simulink model "non_linear"  (R2016a)
settings: Solver=FixedStepAuto  StartTime=0.0  StopTime=300  FixedStep=0.0005  RelTol=1e-3
libraries: simulink x3
settings Model: Creator=mikae  LastModifiedBy=jamie

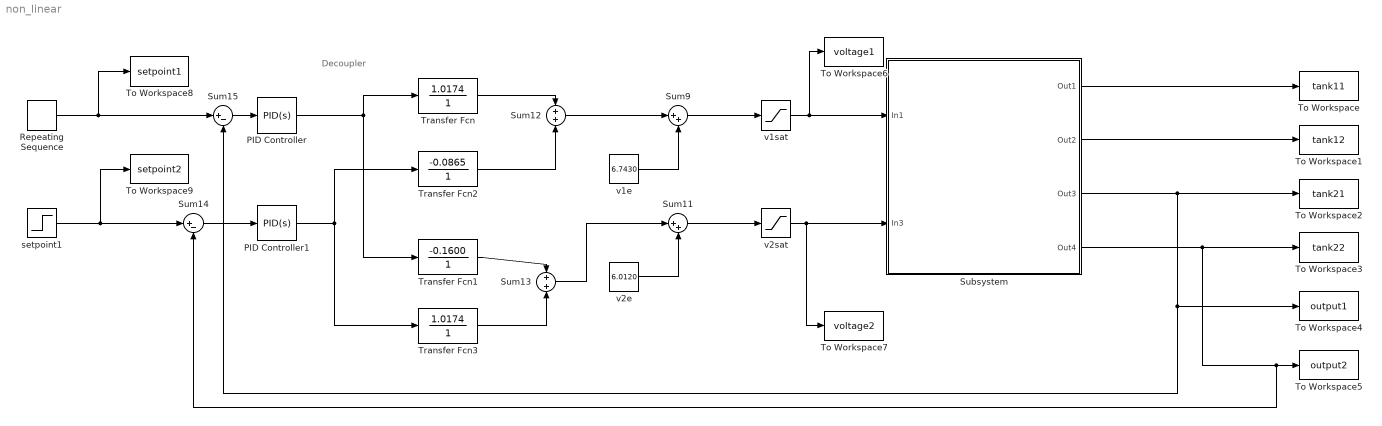
== system non_linear ==
  note: Decoupler
  PID Controller : simulink/Continuous/PID Controller  Controller=PID  TimeDomain=Continuous-time  SampleTime=-1  IntegratorMethod=Forward Euler  FilterMethod=Forward Euler  Form=Ideal  UseFilter=on  ControllerParametersSource=internal  P=1.4351  I=0.0051437  D=10.0105  N=100  InitialConditionSource=internal  InitialConditionForIntegrator=0  InitialConditionForFilter=0  ExternalReset=none  LimitOutput=off  UpperSaturationLimit=inf  LowerSaturationLimit=-inf  LinearizeAsGain=on  AntiWindupMode=none  Kb=1  TrackingMode=off  Kt=1  PParamMin=[]  PParamMax=[]  IParamMin=[]  IParamMax=[]  DParamMin=[]  DParamMax=[]  NParamMin=[]  NParamMax=[]  KbParamMin=[]  KbParamMax=[]  KtParamMin=[]  KtParamMax=[]  POutMin=[]  POutMax=[]  IOutMin=[]  IOutMax=[]  DOutMin=[]  DOutMax=[]  NOutMin=[]  NOutMax=[]  KbOutMin=[]  KbOutMax=[]  KtOutMin=[]  KtOutMax=[]  IntegratorOutMin=[]  IntegratorOutMax=[]  FilterOutMin=[]  FilterOutMax=[]  SumOutMin=[]  SumOutMax=[]  SumI1OutMin=[]  SumI1OutMax=[]  SumI2OutMin=[]  SumI2OutMax=[]  SumI3OutMin=[]  SumI3OutMax=[]  SumDOutMin=[]  SumDOutMax=[]  SaturationOutMin=[]  SaturationOutMax=[]  IntegratorContinuousStateAttributes=''  IntegratorStateMustResolveToSignalObject=off  IntegratorRTWStateStorageClass=Auto  FilterContinuousStateAttributes=''  FilterStateMustResolveToSignalObject=off  FilterRTWStateStorageClass=Auto  DifferentiatorICPrevScaledInput=0  DifferentiatorOutMin=[]  DifferentiatorOutMax=[]
  PID Controller1 : simulink/Continuous/PID Controller  Controller=PID  TimeDomain=Continuous-time  SampleTime=-1  IntegratorMethod=Forward Euler  FilterMethod=Forward Euler  Form=Parallel  UseFilter=on  ControllerParametersSource=internal  P=1.4351  I=0.0051437  D=10.0105  N=100  InitialConditionSource=internal  InitialConditionForIntegrator=0  InitialConditionForFilter=0  ExternalReset=none  LimitOutput=off  UpperSaturationLimit=inf  LowerSaturationLimit=-inf  LinearizeAsGain=on  AntiWindupMode=none  Kb=1  TrackingMode=off  Kt=1  PParamMin=[]  PParamMax=[]  IParamMin=[]  IParamMax=[]  DParamMin=[]  DParamMax=[]  NParamMin=[]  NParamMax=[]  KbParamMin=[]  KbParamMax=[]  KtParamMin=[]  KtParamMax=[]  POutMin=[]  POutMax=[]  IOutMin=[]  IOutMax=[]  DOutMin=[]  DOutMax=[]  NOutMin=[]  NOutMax=[]  KbOutMin=[]  KbOutMax=[]  KtOutMin=[]  KtOutMax=[]  IntegratorOutMin=[]  IntegratorOutMax=[]  FilterOutMin=[]  FilterOutMax=[]  SumOutMin=[]  SumOutMax=[]  SumI1OutMin=[]  SumI1OutMax=[]  SumI2OutMin=[]  SumI2OutMax=[]  SumI3OutMin=[]  SumI3OutMax=[]  SumDOutMin=[]  SumDOutMax=[]  SaturationOutMin=[]  SaturationOutMax=[]  IntegratorContinuousStateAttributes=''  IntegratorStateMustResolveToSignalObject=off  IntegratorRTWStateStorageClass=Auto  FilterContinuousStateAttributes=''  FilterStateMustResolveToSignalObject=off  FilterRTWStateStorageClass=Auto  DifferentiatorICPrevScaledInput=0  DifferentiatorOutMin=[]  DifferentiatorOutMax=[]
  Repeating Sequence : simulink/Sources/Repeating Sequence  rep_seq_t="[1\t1.50000000000000\t2\t2.50000000000000\t3\t3.50000000000000\t4\t4.50000000000000\t5\t5.50000000000000\t6\t6.50000000000000\t7\t7.50000000000000\t8\t8.50000000000000\t9\t9.50000000000000\t10\t10.5000000000000\t11\t11.5000000000000\t12\t12.5000000000000\t13\t13.5000000000000\t14\t14.5000000000000\t15\t15.5000000000000\t16\t16.5000000000000\t17\t17.5000000000000\t18\t18.5000000000000\t19\t19.5000000000000\t20\t20.5000000000000\t21\t21.5000000000000\t22\t22.5000000000000\t23\t23.5000000000000\t24\t24.5000000000000\t25\t25.5000000000000\t26\t26.5000000000000\t27\t27.5000000000000\t28\t28.5000000000000\t29\t29.5000000000000\t30\t30.5000000000000\t31\t31.5000000000000\t32\t32.5000000000000\t33\t33.5000000000000\t34\t34.5000000000000\t35\t35.5000000000000\t36\t36.5000000000000\t37\t37.5000000000000\t38\t38.5000000000000\t39\t39.5000000000000\t40\t40.5000000000000\t41\t41.5000000000000\t42\t42.5000000000000\t43\t43.5000000000000\t44\t44.5000000000000\t45\t45.5000000000000\t46\t46.5000000000000\t47\t47.5000000000000\t48\t48.5000000000000\t49\t49.5000000000000\t50\t50.5000000000000\t51\t51.5000000000000\t52\t52.5000000000000\t53\t53.5000000000000\t54\t54.5000000000000\t55\t55.5000000000000\t56\t56.5000000000000\t57\t57.5000000000000\t58\t58.5000000000000\t59\t59.5000000000000\t60\t60.5000000000000\t61\t61.5000000000000\t62\t62.5000000000000\t63\t63.5000000000000\t64\t64.5000000000000\t65\t65.5000000000000\t66\t66.5000000000000\t67\t67.5000000000000\t68\t68.5000000000000\t69\t69.5000000000000\t70\t70.5000000000000\t71\t71.5000000000000\t72\t72.5000000000000\t73\t73.5000000000000\t74\t74.5000000000000\t75\t75.5000000000000\t76\t76.5000000000000\t77\t77.5000000000000\t78\t78.5000000000000\t79\t79.5000000000000\t80\t80.5000000000000\t81\t81.5000000000000\t82\t82.5000000000000\t83\t83.5000000000000\t84\t84.5000000000000\t85\t85.5000000000000\t86\t86.5000000000000\t87\t87.5000000000000\t88\t88.5000000000000\t89\t89.5000000000000\t90\t90.5000000000000\t91\t91.5000000000000\t92\t92.5000000000000\t93\t93.5000000000000\t94\t94.5000000000000\t95\t95.5000000000000\t96\t96.5000000000000\t97\t97.5000000000000\t98\t98.5000000000000\t99\t99.5000000000000\t100\t100.500000000000\t101\t101.500000000000\t102\t102.500000000000\t103\t103.500000000000\t104\t104.500000000000\t105\t105.500000000000\t106\t106.500000000000\t107\t107.500000000000\t108\t108.500000000000\t109\t109.500000000000\t110\t110.500000000000\t111\t111.500000000000\t112\t112.500000000000\t113\t113.500000000000\t114\t114.500000000000\t115\t115.500000000000\t116\t116.500000000000\t117\t117.500000000000\t118\t118.500000000000\t119\t119.500000000000\t120\t120.500000000000\t121\t121.500000000000\t122\t122.500000000000\t123\t123.500000000000\t124\t124.500000000000\t125\t125.500000000000\t126\t126.500000000000\t127\t127.500000000000\t128\t128.500000000000\t129\t129.500000000000\t130\t130.500000000000\t131\t131.500000000000\t132\t132.500000000000\t133\t133.500000000000\t134\t134.500000000000\t135\t135.500000000000\t136\t136.500000000000\t137\t137.500000000000\t138\t138.500000000000\t139\t139.500000000000\t140\t140.500000000000\t141\t141.500000000000\t142\t142.500000000000\t143\t143.500000000000\t144\t144.500000000000\t145\t145.500000000000\t146\t146.500000000000\t147\t147.500000000000\t148\t148.500000000000\t149\t149.500000000000\t150\t150.500000000000\t151\t151.500000000000\t152\t152.500000000000\t153\t153.500000000000\t154\t154.500000000000\t155\t155.500000000000\t156\t156.500000000000\t157\t157.500000000000\t158\t158.500000000000\t159\t159.500000000000\t160\t160.500000000000\t161\t161.500000000000\t162\t162.500000000000\t163\t163.500000000000\t164\t164.500000000000\t165\t165.500000000000\t166\t166.500000000000\t167\t167.500000000000\t168\t168.500000000000\t169\t169.500000000000\t170\t170.500000000000\t171\t171.500000000000\t172\t172.500000000000\t173\t173.500000000000\t174\t174.500000000000\t175\t175.500000000000\t176\t176.500000000000\t177\t177.500000000000\t178\t178.500000000000\t179\t179.500000000000\t180\t180.500000000000\t181\t181.500000000000\t182\t182.500000000000\t183\t183.500000000000\t184\t184.500000000000\t185\t185.500000000000\t186\t186.500000000000\t187\t187.500000000000\t188\t188.500000000000\t189\t189.500000000000\t190\t190.500000000000\t191\t191.500000000000\t192\t192.500000000000\t193\t193.500000000000\t194\t194.500000000000\t195\t195.500000000000\t196\t196.500000000000\t197\t197.500000000000\t198\t198.500000000000\t199\t199.500000000000\t200\t200.500000000000\t201\t201.500000000000\t202\t202.500000000000\t203\t203.500000000000\t204\t204.500000000000\t205\t205.500000000000\t206\t206.500000000000\t207\t207.500000000000\t208\t208.500000000000\t209\t209.500000000000\t210\t210.500000000000\t211\t211.500000000000\t212\t212.500000000000\t213\t213.500000000000\t214\t214.500000000000\t215\t215.500000000000\t216\t216.500000000000\t217\t217.500000000000\t218\t218.500000000000\t219\t219.500000000000\t220\t220.500000000000\t221\t221.500000000000\t222\t222.500000000000\t223\t223.500000000000\t224\t224.500000000000\t225\t225.500000000000\t226\t226.500000000000\t227\t227.500000000000\t228\t228.500000000000\t229\t229.500000000000\t230\t230.500000000000\t231\t231.500000000000\t232\t232.500000000000\t233\t233.500000000000\t234\t234.500000000000\t235\t235.500000000000\t236\t236.500000000000\t237\t237.500000000000\t238\t238.500000000000\t239\t239.500000000000\t240\t240.500000000000\t241\t241.500000000000\t242\t242.500000000000\t243\t243.500000000000\t244\t244.500000000000\t245\t245.500000000000\t246\t246.500000000000\t247\t247.500000000000\t248\t248.500000000000\t249\t249.500000000000\t250\t250.500000000000]"  rep_seq_y="[2\t2\t2\t2\t2\t2\t2\t2\t2\t2\t2\t2\t2\t2\t2\t2\t2\t2\t2\t2\t2\t2\t2\t2\t2\t2\t2\t2\t2\t2\t2\t2\t2\t2\t2\t2\t2\t2\t2\t2\t2\t2\t2\t2\t2\t2\t2\t2\t2\t2\t2\t2\t2\t2\t2\t2\t2\t2\t2\t2\t2\t2\t2\t2\t2\t2\t2\t2\t2\t2\t2\t2\t2\t2\t2\t2\t2\t2\t2\t2\t2\t2\t2\t2\t2\t2\t2\t2\t2\t2\t2\t2\t2\t2\t2\t2\t2\t2\t2\t2\t2.10800000000000\t2.21600000000000\t2.32400000000000\t2.43200000000000\t2.54000000000000\t2.64800000000000\t2.75600000000000\t2.86400000000000\t2.97200000000000\t3.08000000000000\t3.18800000000000\t3.29600000000000\t3.40400000000000\t3.51200000000000\t3.62000000000000\t3.72800000000000\t3.83600000000000\t3.94400000000000\t4.05200000000000\t4.16000000000000\t4.26800000000000\t4.37600000000000\t4.48400000000000\t4.59200000000000\t4.70000000000000\t4.80800000000000\t4.91600000000000\t5.02400000000000\t5.13200000000000\t5.24000000000000\t5.34800000000000\t5.45600000000000\t5.56400000000000\t5.67200000000000\t5.78000000000000\t5.88800000000000\t5.99600000000000\t6.10400000000000\t6.21200000000000\t6.32000000000000\t6.42800000000000\t6.53600000000000\t6.64400000000000\t6.75200000000000\t6.86000000000000\t6.96800000000000\t7.07600000000000\t7.18400000000000\t7.29200000000000\t7.40000000000000\t7.50800000000000\t7.61600000000000\t7.72400000000000\t7.83200000000000\t7.94000000000000\t8.04800000000000\t8.15600000000000\t8.26400000000000\t8.37200000000000\t8.48000000000000\t8.58800000000000\t8.69600000000000\t8.80400000000000\t8.91200000000000\t9.02000000000000\t9.12800000000000\t9.23600000000000\t9.34400000000000\t9.45200000000000\t9.56000000000000\t9.66800000000000\t9.77600000000000\t9.88400000000000\t9.99200000000000\t10.1000000000000\t10.2080000000000\t10.3160000000000\t10.4240000000000\t10.5320000000000\t10.6400000000000\t10.7480000000000\t10.8560000000000\t10.9640000000000\t11.0720000000000\t11.1800000000000\t11.2880000000000\t11.3960000000000\t11.5040000000000\t11.6120000000000\t11.7200000000000\t11.8280000000000\t11.9360000000000\t12.0440000000000\t12.1520000000000\t12.2600000000000\t12.3680000000000\t12.4760000000000\t12.5840000000000\t12.6920000000000\t12.8000000000000\t12.9080000000000\t13.0160000000000\t13.1240000000000\t13.2320000000000\t13.3400000000000\t13.4480000000000\t13.5560000000000\t13.6640000000000\t13.7720000000000\t13.8800000000000\t13.9880000000000\t14.0960000000000\t14.2040000000000\t14.3120000000000\t14.4200000000000\t14.5280000000000\t14.6360000000000\t14.7440000000000\t14.8520000000000\t14.9600000000000\t15.0680000000000\t15.1760000000000\t15.2840000000000\t15.3920000000000\t15.5000000000000\t15.5000000000000\t15.5000000000000\t15.5000000000000\t15.5000000000000\t15.5000000000000\t15.5000000000000\t15.5000000000000\t15.5000000000000\t15.5000000000000\t15.5000000000000\t15.5000000000000\t15.5000000000000\t15.5000000000000\t15.5000000000000\t15.5000000000000\t15.5000000000000\t15.5000000000000\t15.5000000000000\t15.5000000000000\t15.5000000000000\t15.5000000000000\t15.5000000000000\t15.5000000000000\t15.5000000000000\t15.5000000000000\t15.5000000000000\t15.5000000000000\t15.5000000000000\t15.5000000000000\t15.5000000000000\t15.5000000000000\t15.5000000000000\t15.5000000000000\t15.5000000000000\t15.5000000000000\t15.5000000000000\t15.5000000000000\t15.5000000000000\t15.5000000000000\t15.5000000000000\t15.5000000000000\t15.5000000000000\t15.5000000000000\t15.5000000000000\t15.5000000000000\t15.5000000000000\t15.5000000000000\t15.5000000000000\t15.5000000000000\t15.5000000000000\t15.5000000000000\t15.5000000000000\t15.5000000000000\t15.5000000000000\t15.5000000000000\t15.5000000000000\t15.5000000000000\t15.5000000000000\t15.5000000000000\t15.5000000000000\t15.5000000000000\t15.5000000000000\t15.5000000000000\t15.5000000000000\t15.5000000000000\t15.5000000000000\t15.5000000000000\t15.5000000000000\t15.5000000000000\t15.5000000000000\t15.5000000000000\t15.5000000000000\t15.5000000000000\t15.5000000000000\t15.5000000000000\t15.5000000000000\t15.5000000000000\t15.5000000000000\t15.5000000000000\t15.5000000000000\t15.5000000000000\t15.5000000000000\t15.5000000000000\t15.5000000000000\t15.5000000000000\t15.5000000000000\t15.5000000000000\t15.5000000000000\t15.5000000000000\t15.5000000000000\t15.6180000000000\t15.7360000000000\t15.8540000000000\t15.9720000000000\t16.0900000000000\t16.2080000000000\t16.3260000000000\t16.4440000000000\t16.5620000000000\t16.6800000000000\t16.7980000000000\t16.9160000000000\t17.0340000000000\t17.1520000000000\t17.2700000000000\t17.3880000000000\t17.5060000000000\t17.6240000000000\t17.7420000000000\t17.8600000000000\t17.9780000000000\t18.0960000000000\t18.2140000000000\t18.3320000000000\t18.4500000000000\t18.5680000000000\t18.6860000000000\t18.8040000000000\t18.9220000000000\t19.0400000000000\t19.1580000000000\t19.2760000000000\t19.3940000000000\t19.5120000000000\t19.6300000000000\t19.7480000000000\t19.8660000000000\t19.9840000000000\t20.1020000000000\t20.2200000000000\t20.3380000000000\t20.4560000000000\t20.5740000000000\t20.6920000000000\t20.8100000000000\t20.9280000000000\t21.0460000000000\t21.1640000000000\t21.2820000000000\t21.4000000000000\t21.5180000000000\t21.6360000000000\t21.7540000000000\t21.8720000000000\t21.9900000000000\t21.8850000000000\t21.7700000000000\t21.6550000000000\t21.5400000000000\t21.4250000000000\t21.3100000000000\t21.1950000000000\t21.0800000000000\t20.9650000000000\t20.8500000000000\t20.7350000000000\t20.6200000000000\t20.5050000000000\t20.3900000000000\t20.2750000000000\t20.1600000000000\t20.0450000000000\t19.9300000000000\t19.8150000000000\t19.7000000000000\t19.5850000000000\t19.4700000000000\t19.3550000000000\t19.2400000000000\t19.1250000000000\t19.0100000000000\t18.8950000000000\t18.7800000000000\t18.6650000000000\t18.5500000000000\t18.4350000000000\t18.3200000000000\t18.2050000000000\t18.0900000000000\t17.9750000000000\t17.8600000000000\t17.7450000000000\t17.6300000000000\t17.5150000000000\t17.4000000000000\t17.2850000000000\t17.1700000000000\t17.0550000000000\t16.9400000000000\t16.8250000000000\t16.7100000000000\t16.5950000000000\t16.4800000000000\t16.3650000000000\t16.2500000000000\t16.1350000000000\t16.0200000000000\t15.9050000000000\t15.7900000000000\t15.6750000000000\t15.5600000000000\t15.4450000000000\t15.3300000000000\t15.2150000000000\t15.1000000000000\t14.9850000000000\t14.8700000000000\t14.7550000000000\t14.6400000000000\t14.5250000000000\t14.4100000000000\t14.2950000000000\t14.1800000000000\t14.0650000000000\t13.9500000000000\t13.8350000000000\t13.7200000000000\t13.6050000000000\t13.4900000000000\t13.3750000000000\t13.2600000000000\t13.1450000000000\t13.0300000000000\t12.9150000000000\t12.8000000000000\t12.6850000000000\t12.5700000000000\t12.4550000000000\t12.3400000000000\t12.2250000000000\t12.1100000000000\t11.9950000000000\t11.8800000000000\t11.7650000000000\t11.6500000000000\t11.5350000000000\t11.4200000000000\t11.3050000000000\t11.1900000000000\t11.0750000000000\t10.9600000000000\t10.8450000000000\t10.7300000000000\t10.6150000000000\t10.5000000000000\t10.3850000000000\t10.2700000000000\t10.1550000000000\t10.0400000000000\t9.92500000000000\t9.81000000000000\t9.69500000000000\t9.58000000000000\t9.46500000000000\t9.35000000000000\t9.23500000000000\t9.12000000000000\t9.00500000000000\t8.89000000000000\t8.77500000000000\t8.66000000000000\t8.54500000000000\t8.43000000000000\t8.31500000000000\t8.20000000000000\t8.08500000000000\t7.97000000000000\t7.85500000000000\t7.74000000000000\t7.62500000000000\t7.51000000000000\t7.39500000000000\t7.28000000000000\t7.16500000000000\t7.05000000000000]"
  Subsystem : Subsystem
  Sum11 : Sum  Inputs=|++
  Sum12 : Sum
  Sum13 : Sum
  Sum14 : Sum  Inputs=|+-
  Sum15 : Sum  Inputs=|+-
  Sum9 : Sum  Inputs=|++
  To Workspace : ToWorkspace  VariableName=tank11  SaveFormat=Timeseries  SampleTime=-1
  To Workspace1 : ToWorkspace  VariableName=tank12  SaveFormat=Timeseries  SampleTime=-1
  To Workspace2 : ToWorkspace  VariableName=tank21  SaveFormat=Timeseries  SampleTime=-1
  To Workspace3 : ToWorkspace  VariableName=tank22  SaveFormat=Timeseries  SampleTime=-1
  To Workspace4 : ToWorkspace  VariableName=output1  SaveFormat=Timeseries  SampleTime=-1
  To Workspace5 : ToWorkspace  VariableName=output2  SaveFormat=Timeseries  SampleTime=-1
  To Workspace6 : ToWorkspace  VariableName=voltage1  SaveFormat=Timeseries  SampleTime=-1
  To Workspace7 : ToWorkspace  VariableName=voltage2  SaveFormat=Timeseries  SampleTime=-1
  To Workspace8 : ToWorkspace  VariableName=setpoint1  SaveFormat=Timeseries  SampleTime=-1
  To Workspace9 : ToWorkspace  VariableName=setpoint2  SaveFormat=Timeseries  SampleTime=-1
  Transfer Fcn : TransferFcn  Numerator=[1.0174]  Denominator=[1]
  Transfer Fcn1 : TransferFcn  Numerator=[-0.1600]  Denominator=[1]
  Transfer Fcn2 : TransferFcn  Numerator=[-0.0865]  Denominator=[1]
  Transfer Fcn3 : TransferFcn  Numerator=[1.0174]  Denominator=[1]
  setpoint1 : Step  Before=22.5  After=26.55  SampleTime=0
  v1e : Constant  Value=6.7430
  v1sat : Saturate  UpperLimit=12  LowerLimit=0
  v2e : Constant  Value=6.0120
  v2sat : Saturate  UpperLimit=12  LowerLimit=0
  wires:
  Sum9/1 -> v1sat/1
  v1e/1 -> Sum9/2
  PID Controller/1 -> Transfer Fcn/1, Transfer Fcn1/1
  PID Controller1/1 -> Transfer Fcn3/1, Transfer Fcn2/1
  Transfer Fcn3/1 -> Sum13/2
  Transfer Fcn1/1 -> Sum13/1
  Transfer Fcn2/1 -> Sum12/2
  Transfer Fcn/1 -> Sum12/1
  Sum12/1 -> Sum9/1
  Sum11/1 -> v2sat/1
  Sum13/1 -> Sum11/1
  v2e/1 -> Sum11/2
  setpoint1/1 -> To Workspace9/1, Sum14/1
  Subsystem/4(Out4) -> Sum14/2, To Workspace5/1, To Workspace3/1
  Repeating Sequence/1 -> To Workspace8/1, Sum15/1
  Subsystem/3(Out3) -> Sum15/2, To Workspace4/1, To Workspace2/1
  Sum15/1 -> PID Controller/1
  Sum14/1 -> PID Controller1/1
  v1sat/1 -> To Workspace6/1, Subsystem/1(In1)
  v2sat/1 -> To Workspace7/1, Subsystem/2(In3)
  Subsystem/1(Out1) -> To Workspace/1
  Subsystem/2(Out2) -> To Workspace1/1

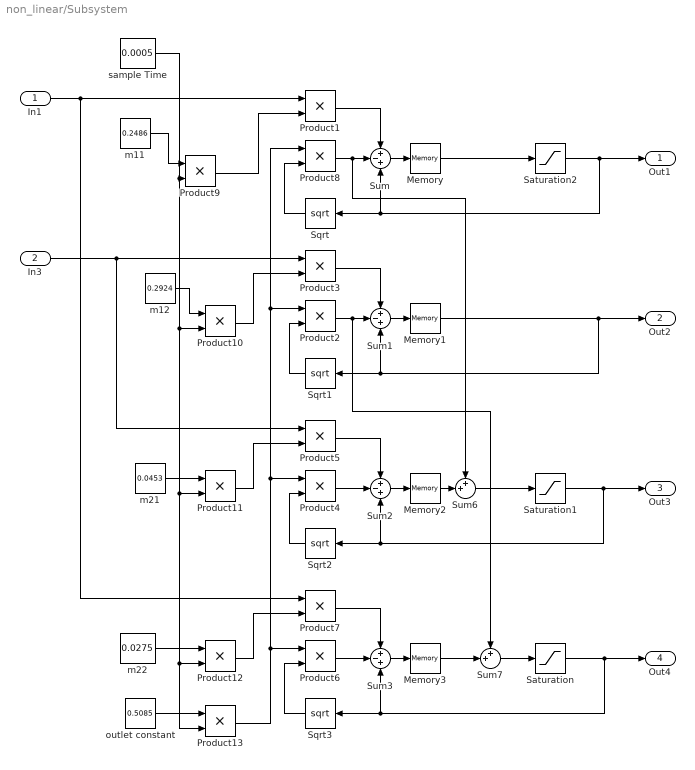
== system non_linear/Subsystem ==
  In1 : Inport
  In3 : Inport  Port=2
  Memory{,1..3} (4 alike) : Memory
  Product{1..13} (13 alike) : Product
  Saturation : Saturate  UpperLimit=30  LowerLimit=0
  Saturation1 : Saturate  UpperLimit=30  LowerLimit=0
  Saturation2 : Saturate  UpperLimit=30  LowerLimit=0
  Sqrt{,1..3} (4 alike) : Sqrt  SaturateOnIntegerOverflow=on
  Sum{,1..3} (4 alike) : Sum  Inputs=+-+
  Sum6 : Sum  Inputs=++|
  Sum7 : Sum  Inputs=++|
  m11 : Constant  Value=0.2486
  m12 : Constant  Value=0.2924
  m21 : Constant  Value=0.0453
  m22 : Constant  Value=0.0275
  outlet constant : Constant  Value=0.5085
  sample Time : Constant  Value=0.0005
  Out1 : Outport
  Out2 : Outport  Port=2
  Out3 : Outport  Port=3
  Out4 : Outport  Port=4
  wires:
  Sum6/1 -> Saturation1/1
  Memory1/1 -> Out2/1, Sum1/3, Sqrt1/1
  Memory/1 -> Saturation2/1
  Sum7/1 -> Saturation/1
  Product13/1 -> Product6/1, Product4/1, Product2/1, Product8/1
  Product9/1 -> Product1/2
  Product3/1 -> Sum1/1
  Product1/1 -> Sum/1
  Product5/1 -> Sum2/1
  Product7/1 -> Sum3/1
  In1/1 -> Product7/1, Product1/1
  Sum2/1 -> Memory2/1
  Product2/1 -> Sum7/1, Sum1/2
  Memory2/1 -> Sum6/2
  Sum3/1 -> Memory3/1
  In3/1 -> Product5/1, Product3/1
  Sqrt/1 -> Product8/2
  Sqrt2/1 -> Product4/2
  Sum/1 -> Memory/1
  Sqrt3/1 -> Product6/2
  Product8/1 -> Sum6/1, Sum/2
  Sum1/1 -> Memory1/1
  Sqrt1/1 -> Product2/2
  Product4/1 -> Sum2/2
  Product6/1 -> Sum3/2
  Memory3/1 -> Sum7/2
  Saturation/1 -> Out4/1, Sum3/3, Sqrt3/1
  Saturation1/1 -> Out3/1, Sqrt2/1, Sum2/3
  Saturation2/1 -> Out1/1, Sum/3, Sqrt/1
  m11/1 -> Product9/1
  m12/1 -> Product10/1
  Product10/1 -> Product3/2
  Product11/1 -> Product5/2
  m21/1 -> Product11/1
  Product12/1 -> Product7/2
  m22/1 -> Product12/1
  outlet constant/1 -> Product13/1
  sample Time/1 -> Product9/2, Product11/2, Product12/2, Product13/2, Product10/2
